simulink model "week1problem1_2019a"  (R2019a)
settings: Solver=VariableStepAuto  StartTime=0.0  StopTime=50  RelTol=1e-3
model workspace (MAT data in the model file):
  b = 50
  k1 = 50
  k12 = 0
  m1 = 100
  m2 = 0
settings Model: OrderedModelArguments=off  Creator=rutvi  LastModifiedBy=rutvi

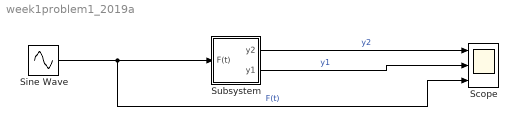
== system week1problem1_2019a ==
  Scope : Scope  NumInputPorts=3
  Sine Wave : Sin  Amplitude=2  Frequency=10  SampleTime=0
  Subsystem : Subsystem  mask{m2=60.0, k12=300.0}
  wires:
  Subsystem/1(y2) -> Scope/1  "y2"
  Subsystem/2(y1) -> Scope/2  "y1"
  Sine Wave/1 -> Scope/3, Subsystem/1(F(t))  "F(t)"

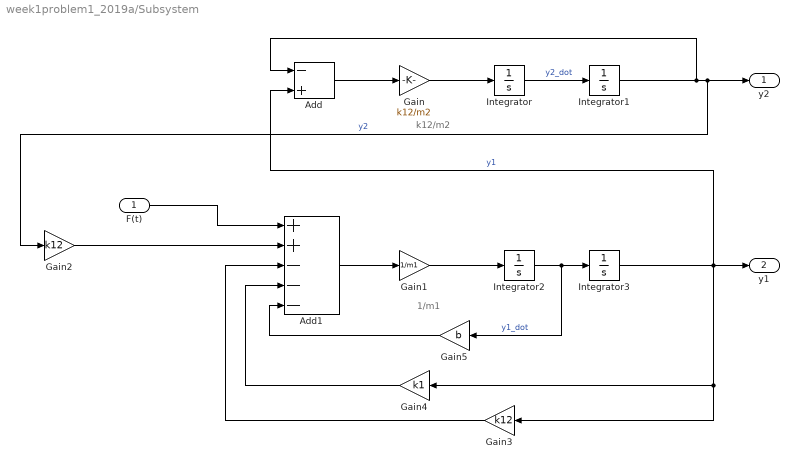
== system week1problem1_2019a/Subsystem ==
  note: 1/m1
  note: k12/m2
  F(t) : Inport
  Add : Sum  Inputs=-+
  Add1 : Sum  Inputs=++---
  Gain : Gain  Gain=k12/m2
  Gain1 : Gain  Gain=1/m1
  Gain2 : Gain  Gain=k12
  Gain3 : Gain  Gain=k12
  Gain4 : Gain  Gain=k1
  Gain5 : Gain  Gain=b
  Integrator{,1..3} (4 alike) : Integrator
  y2 : Outport
  y1 : Outport  Port=2
  wires:
  Add/1 -> Gain/1
  Gain/1 -> Integrator/1
  Integrator/1 -> Integrator1/1  "y2_dot"
  Integrator1/1 -> Add/1, Gain2/1, y2/1  "y2"
  F(t)/1 -> Add1/1
  Add1/1 -> Gain1/1
  Gain1/1 -> Integrator2/1
  Integrator2/1 -> Gain5/1, Integrator3/1  "y1_dot"
  Integrator3/1 -> Add/2, y1/1, Gain4/1, Gain3/1  "y1"
  Gain2/1 -> Add1/2
  Gain3/1 -> Add1/3
  Gain4/1 -> Add1/4
  Gain5/1 -> Add1/5
